simulink model "adaptive_control"  (R2024a)
settings: Solver=FixedStepAuto  StartTime=0.0  StopTime=10  FixedStep=1e-3  RelTol=1e-3
settings Model: Creator=erhan  LastModifiedBy=erhan

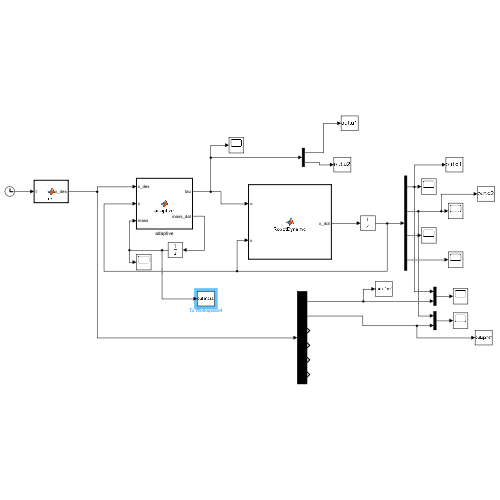
[thumbnail: Simulink's stored preview of the top-level diagram]
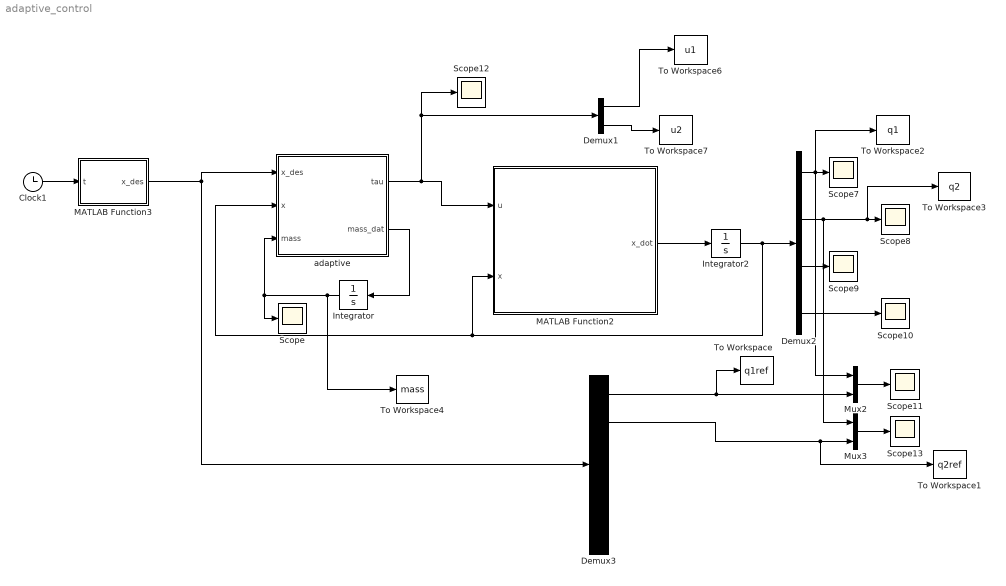
== system adaptive_control ==
  Clock1 : Clock
  Demux1 : Demux  Outputs=2
  Demux2 : Demux
  Demux3 : Demux  Outputs=6
  Integrator : Integrator  InitialCondition=[0;0]
  Integrator2 : Integrator  InitialCondition=[0;0;0;0]
  MATLAB Function2 : MATLAB Function  TreatAsAtomicUnit=on
  MATLAB Function3 : MATLAB Function  TreatAsAtomicUnit=on
  Mux2 : Mux  Inputs=2
  Mux3 : Mux  Inputs=2
  Scope{,7..13} (8 alike) : Scope
  To Workspace : ToWorkspace  VariableName=q1ref  SaveFormat=Timeseries  SampleTime=-1
  To Workspace1 : ToWorkspace  VariableName=q2ref  SaveFormat=Timeseries  SampleTime=-1
  To Workspace2 : ToWorkspace  VariableName=q1  SaveFormat=Timeseries  SampleTime=-1
  To Workspace3 : ToWorkspace  VariableName=q2  SaveFormat=Timeseries  SampleTime=-1
  To Workspace4 : ToWorkspace  VariableName=mass  SaveFormat=Timeseries  SampleTime=-1
  To Workspace6 : ToWorkspace  VariableName=u1  SaveFormat=Timeseries  SampleTime=-1
  To Workspace7 : ToWorkspace  VariableName=u2  SaveFormat=Timeseries  SampleTime=-1
  adaptive : MATLAB Function  TreatAsAtomicUnit=on
  wires:
  Mux3/1 -> Scope13/1
  Demux3/2 -> To Workspace1/1, Mux3/2
  Demux3/1 -> To Workspace/1, Mux2/2
  Mux2/1 -> Scope11/1
  Clock1/1 -> MATLAB Function3/1(t)
  MATLAB Function3/1(x_des) -> adaptive/1(x_des), Demux3/1
  Demux2/4 -> Scope10/1
  Demux2/3 -> Scope9/1
  Demux2/2 -> Mux3/1, To Workspace3/1, Scope8/1
  Demux2/1 -> Mux2/1, To Workspace2/1, Scope7/1
  Integrator2/1 -> MATLAB Function2/2(x), adaptive/2(x), Demux2/1
  MATLAB Function2/1(x_dot) -> Integrator2/1
  adaptive/1(tau) -> Demux1/1, Scope12/1, MATLAB Function2/1(u)
  adaptive/2(mass_dat) -> Integrator/1
  Integrator/1 -> To Workspace4/1, adaptive/3(mass), Scope/1
  Demux1/1 -> To Workspace6/1
  Demux1/2 -> To Workspace7/1

== matlab function adaptive_control/MATLAB Function2 ==
  data: u input; x_dot output; x input
function x_dot = RobotDynamic(u,x)
% Parametreler
m1=0.8; m2=2;
L1=1; L2=1;
g=9.81;

% --- M (Atalet) Matrisi ---
M11 = (m2*(2*L1^2 + 2*L2^2 + 4*L1*L2*cos(x(2))))/2 + L1^2*m1;
M12 = L2*m2*(L2 + L1*cos(x(2)));
M21 = M12;
M22 = L2^2*m2;

% --- C (Coriolis/Merkezkaç) Vektörü ---
C1 = -L1*L2*x(4)*m2*sin(x(2))*(2*x(3) + x(4));
C2 = L1*L2*x(3)^2*m2*sin(x(2));

% --- G (Yerçekimi) Vektörü ---
G1 = g*m2*(L2*cos(x(1) + x(2)) + L1*cos(x(1))) + L1*g*m1*cos(x(1));
G2 = L2*g*m2*cos(x(1) + x(2));


% N (Nonlinear Terms)
N1 = G1 + C1;
N2 = G2 + C2;

% --- MATRİS TERSİ (Inverse Matrix) HESABI ---
% Determinant
det = M11*M22 - M12*M21;

% HATA BURADAYDI (Düzeltildi)
MI11 = M22/det;
MI12 = -M12/det;
MI21 = -M21/det;  % Eksikti, eklendi.
MI22 = M11/det;   % MI11 yerine MI22 yazildi.

% Giriş Torkları
tau1 = u(1);
tau2 = u(2);

% --- İVMELERİN HESAPLANMASI ---
% Denklem: ddq = inv(M) * (tau - N)
% q(3) -> ddq1
% q(4) -> ddq2

q = zeros(4,1);
q(1) = x(3); % dq1
q(2) = x(4); % dq2

% Matris çarpımı (Manuel):
% ddq1 = MI11*(tau1 - N1) + MI12*(tau2 - N2)
q(3) = MI11*(tau1 - N1) + MI12*(tau2 - N2);

% ddq2 = MI21*(tau1 - N1) + MI22*(tau2 - N2)
q(4) = MI21*(tau1 - N1) + MI22*(tau2 - N2);

x_dot = q;
end

== matlab function adaptive_control/MATLAB Function3 ==
  data: t input; x_des output
function x_des = ref(t)


period = 2;
amp1 = 0.1;
amp2 = 0.1;
fact = 2*pi/period;
sinf = sin(fact*t);
cosf = cos(fact*t);
qd = [amp1*sinf amp2*cosf];
qdp = fact*[amp1*cosf -amp2*sinf];
qdpp = -fact^2*qd;
x_des = [qd qdp qdpp]';

end

== matlab function adaptive_control/adaptive ==
  data: tau output; x_des input; mass_dat output; x input; mass input
function [tau,mass_dat] = adaptive(x_des, x,mass)

% Robust_PD_Gravity_Control: Robot için sağlam PD yerçekimi kontrolcüsü uygular.
% Bu fonksiyon, kontrol teorisindeki tau = Kv*r + G - v yasasını esas alır.
% Girişler:
% x_des     : [6x1] (qd, qd_dot, qd_dot_dot) vektörü
% x         : [4x1] (q, dq) anlık durum vektörü


%% --- PARAMETRELER VE KAZANÇLAR ---
% Kol Parametreleri (m1, m2, a1, a2)
% Parametreler
m1=0.8; m2=2.3;
a1=1; a2=1;
g=9.81;

% Kontrol Kazançları ve Filtreleme
Kv = 30* eye(2);               % Hız Kazanç Matrisi (Kd = Kv)
lam =9;               % Filtreleme Matrisi (Lambda)
                      % Sınırlayıcı Katman Genişliği (epsilon)
gam =0.1*eye(2);

e1 =  x_des(1) - x(1);
e2 =  x_des(2) - x(2);
ep1 = x_des(3) - x(3);
ep2 = x_des(4) - x(4);
r1 = ep1 + lam*e1;
r2 = ep2 + lam*e2;
r=[r1;r2];

qr1d = x_des(3) + lam*e1;
qr2d = x_des(4) + lam*e2;
qr1dd = x_des(5) + lam*ep1;
qr2dd = x_des(6) + lam*ep2;
W=ones(2,2);
W(1,1) = a1*g*cos(x(1)) + a1*a1*qr1dd;
W(1,2) = g*(a2*cos(x(1)+x(2))+a1*cos(x(1))) + a1*a2*sin(x(2))*(-x(4)*qr1d + qr2d*(x(3)+x(4))) + a2*(a2+a1*cos(x(2)))*qr2dd + qr1dd*(a1*a1 + a2*a2 + 2*a1*a2*cos(x(2)));
W(2,1) = 0;
W(2,2) = a2*g*cos(x(1)+x(2)) + a1*a2*sin(x(2))*x(3)*qr1d + a2*a2*qr2dd + a2*(a2+a1+cos(x(2)))*qr1dd;


tau = Kv*r + W*[mass(1);mass(2)];
tau1 = tau(1);
tau2=tau(2);
phi_dot = gam*W'*r;
mass1_dat = phi_dot(1);
mass2_dat = phi_dot(2);
mass_dat=[mass1_dat;mass2_dat];




end
